simulink model "c28069pmsmfoc_cla"  (R2021b)
settings: Solver=FixedStepDiscrete  StartTime=0.0  StopTime=inf  RelTol=1e-3  EnableMultiTasking=on
PreLoadFcn:
  | c28069pmsmfoc_data;
model workspace (MAT data in the model file):
  encoderResolution = 2000
  hallOffset = '0.5'
  indexOffset = 850
  polePairs = '4'
values from neighbouring files (symbols this model uses):
  Hall_position_offset = 0.57    [c28027pmsmfoc_data.m]    (also in c28035pmsmfoc_data.m; c28035pmsmfoc_data_cla.m; c28069pmsmfoc_data.m)
  PWM_Counter_Period = CPU_frequency/PWM_frequency/2    (= 1500)    [c28027pmsmfoc_data.m]    (also in c28035pmsmfoc_data.m; c28035pmsmfoc_data_cla.m = 2500; c28069pmsmfoc_data.m = 2250)
  Speed_per_unit_scaler = 1200    [c28027pmsmfoc_data.m]    (also in c28035pmsmfoc_data.m; c28035pmsmfoc_data_cla.m = 600; c28069pmsmfoc_data.m)
  Speed_rpm_scaler = 60*CPU_frequency/Pole_pairs/2    (= 450000000)    [c28027pmsmfoc_data.m]    (also in c28035pmsmfoc_data.m; c28035pmsmfoc_data_cla.m; c28069pmsmfoc_data.m = 675000000)
undefined symbols (not defined in the file or in its folder): codertarget, Down, GPTRIP1SEL, GPTRIP2SEL, TZ1, TZ2, Up
libraries: idelinklib_common x12, c2802xlib x7, tiiqmathlib x7, hall_sensor_lib x7, c280xlib x3, c2803xlib x2, simulink x2, etargetslib x2, demo_controls x1, c2806xlib x1, c2000lib x1
(part 1 of 3)
settings Model: Creator=The MathWorks, Inc.  LastModifiedBy=The MathWorks, Inc.
settings SolverCC: AlgebraicLoopSolver=TrustRegion
settings DataIOCC: LimitDataPoints=on  SaveFormat=Array  SaveOutput=off  SaveTime=off  ReturnWorkspaceOutputs=off
settings OptimizationCC: DefaultParameterBehavior=Inlined  DefaultUnderspecifiedDataType=single  InlineInvariantSignals=on  BufferReuse=off  ExpressionDepthLimit=2147483647  InitFltsAndDblsToZero=on  NoFixptDivByZeroProtection=on  EfficientFloat2IntCast=on  EfficientMapNaN2IntZero=off  LifeSpan=Inf  MaxStackSize=512  EfficientTunableParamExpr=on
settings DebuggingCC: ReadBeforeWriteMsg=DisableAll  WriteAfterWriteMsg=DisableAll  WriteAfterReadMsg=DisableAll  AlgebraicLoopMsg=error  ArtificialAlgebraicLoopMsg=error  CheckSSInitialOutputMsg=off  UnderspecifiedInitializationDetection=Classic  MergeDetectMultiDrivingBlocksExec=none  SignalResolutionControl=TryResolveAllWithWarning  SolverPrmCheckMsg=warning  InheritedTsInSrcMsg=none  MultiTaskDSMMsg=none  MultiTaskCondExecSysMsg=none  TasksWithSamePriorityMsg=none  SigSpecEnsureSampleTimeMsg=none  IntegerOverflowMsg=none  ParameterPrecisionLossMsg=none  FcnCallInpInsideContextMsg=warning  AllowSymbolicDim=off  StateNameClashWarn=warning  SFUnexpectedBacktrackingDiag=warning  SFNoUnconditionalDefaultTransitionDiag=warning  SFExecutionAtInitializationDiag=none  SFMachineParentedDataDiag=warning  IntegerSaturationMsg=none  ArithmeticOperatorsInVariantConditions=warning
settings HardwareCC: ProdBitPerChar=16  ProdBitPerInt=16  ProdBitPerPointer=32  ProdBitPerSizeT=32  ProdBitPerPtrDiffT=32  ProdLargestAtomicInteger=Integer  ProdLargestAtomicFloat=None  ProdWordSize=16  ProdHWDeviceType=Texas Instruments->C2000  TargetBitPerChar=16  TargetBitPerInt=16  TargetBitPerPointer=16  TargetLargestAtomicInteger=Integer  TargetIntDivRoundTo=Zero  TargetEndianess=LittleEndian  TargetWordSize=16  TargetHWDeviceType=TI C2000
settings ModelReferenceCC: PropagateSignalLabelsOutOfModel=off
settings SFSimCC: SimUseLocalCustomCode=off  MATLABDynamicMemAlloc=off  CustomCodeUndefinedFunction=UseInterfaceOnly
settings RTWCC: Description=Embedded Coder  SystemTargetFile=ert.tlc  HardwareBoard=TI Piccolo F2806x  TemplateMakefile=ert_default_tmf  GenerateReport=on  RTWUseLocalCustomCode=off  Toolchain=Texas Instruments Code Composer Studio (C2000)  BuildConfiguration=Debug  IncludeHyperlinkInReport=on  LaunchReport=on  GenerateTraceInfo=on  GenerateTraceReport=on  GenerateTraceReportSl=on  GenerateTraceReportSf=on  GenerateTraceReportEml=on
settings CodeAppCC: IgnoreCustomStorageClasses=off  CustomSymbolStrType=$N$R$M  StateflowObjectComments=on  InternalIdentifier=Classic
settings ERTTargetCC: CodeReplacementLibrary=TI C28x  MultiwordLength=2048  ExtModeStaticAllocSize=2048  ConvertIfToSwitch=off  SuppressUnreachableDefaultCases=off
settings ConfigComp: CovMetricSettings=dw  CovSaveCumulativeToWorkspaceVar=on  CovSaveSingleToWorkspaceVar=on  CovExternalEMLEnable=off  CovSFcnEnable=off

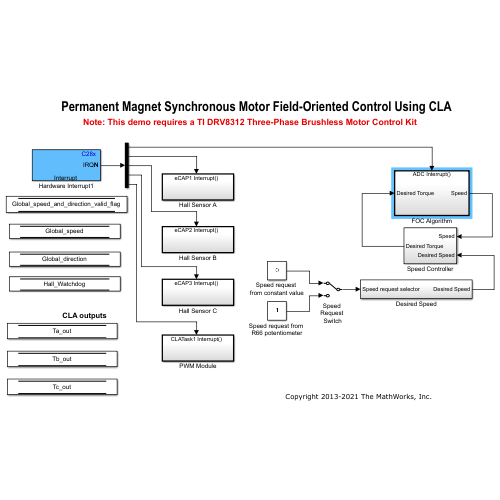
[thumbnail: Simulink's stored preview of the top-level diagram]
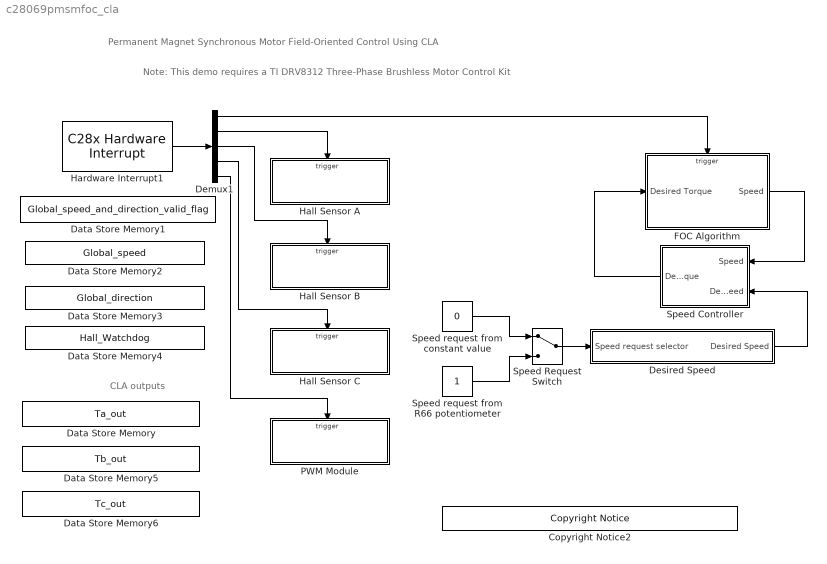
== system c28069pmsmfoc_cla ==
  note: CLA outputs
  note: Note: This demo requires a TI DRV8312 Three-Phase Brushless Motor Control Kit
  note: Permanent Magnet Synchronous Motor Field-Oriented Control Using CLA
  Copyright Notice2 : demo_controls/Copyright Notice  year=2013  prod=tic2000
      settings: SourceProductBaseCode=ME
  Data Store Memory : DataStoreMemory  DataStoreName=Ta_out  ReadBeforeWriteMsg=warning  WriteAfterWriteMsg=warning  WriteAfterReadMsg=warning  EmbeddedSignalClassName=tic2000demospkg.Signal  ShowAdditionalParam=off  OutDataTypeStr=single
  Data Store Memory1 : DataStoreMemory  DataStoreName=Global_speed_and_direction_valid_flag  ReadBeforeWriteMsg=warning  WriteAfterWriteMsg=warning  WriteAfterReadMsg=warning  ShowAdditionalParam=off  OutDataTypeStr=uint16
  Data Store Memory2 : DataStoreMemory  DataStoreName=Global_speed  ReadBeforeWriteMsg=warning  WriteAfterWriteMsg=warning  WriteAfterReadMsg=warning  ShowAdditionalParam=off  OutDataTypeStr=uint32
  Data Store Memory3 : DataStoreMemory  DataStoreName=Global_direction  ReadBeforeWriteMsg=warning  WriteAfterWriteMsg=warning  WriteAfterReadMsg=warning  ShowAdditionalParam=off  OutDataTypeStr=uint16
  Data Store Memory4 : DataStoreMemory  DataStoreName=Hall_Watchdog  ReadBeforeWriteMsg=warning  WriteAfterWriteMsg=warning  WriteAfterReadMsg=warning  InitialValue=65535  ShowAdditionalParam=off  OutDataTypeStr=uint16
  Data Store Memory5 : DataStoreMemory  DataStoreName=Tb_out  ReadBeforeWriteMsg=warning  WriteAfterWriteMsg=warning  WriteAfterReadMsg=warning  EmbeddedSignalClassName=tic2000demospkg.Signal  ShowAdditionalParam=off  OutDataTypeStr=single
  Data Store Memory6 : DataStoreMemory  DataStoreName=Tc_out  ReadBeforeWriteMsg=warning  WriteAfterWriteMsg=warning  WriteAfterReadMsg=warning  EmbeddedSignalClassName=tic2000demospkg.Signal  ShowAdditionalParam=off  OutDataTypeStr=single
  Demux1 : Demux  Outputs=5
  Desired Speed : Subsystem
  FOC Algorithm : Subsystem
  Hall Sensor A : Subsystem  TreatAsAtomicUnit=on
  Hall Sensor B : Subsystem  TreatAsAtomicUnit=on
  Hall Sensor C : Subsystem  TreatAsAtomicUnit=on
  Hardware Interrupt1 : c2000lib/Scheduling/C28x Hardware Interrupt  irqnumbers=[1 4 4 4 11]  pienumbers=[1 1 2 3 1]  irqpriorities=[30 25 25 25 27]  irqpreempts=[1 0 0 0 1]  showinput=off  dspchiptype=C280X
      settings: SourceProductBaseCode=TIC2000
  PWM Module : Subsystem  TreatAsAtomicUnit=on
  Speed Request Switch : ManualSwitch
  Speed Controller : Subsystem
  Speed request from constant value : Constant  Value=0  OutDataTypeStr=uint16
  Speed request from R66 potentiometer : Constant  OutDataTypeStr=uint16
  wires:
  Hardware Interrupt1/1 -> Demux1/1
  Demux1/1 -> FOC Algorithm/Trigger
  Demux1/2 -> Hall Sensor A/Trigger
  Demux1/3 -> Hall Sensor B/Trigger
  Demux1/4 -> Hall Sensor C/Trigger
  FOC Algorithm/1(Speed) -> Speed Controller/1(Speed)
  Speed Controller/1(Desired Torque) -> FOC Algorithm/1(Desired Torque)
  Desired Speed/1(Desired Speed) -> Speed Controller/2(Desired Speed)
  Speed Request Switch/1 -> Desired Speed/1(Speed request selector)
  Speed request from constant value/1 -> Speed Request Switch/1
  Speed request from R66 potentiometer/1 -> Speed Request Switch/2
  Demux1/5 -> PWM Module/Trigger

== system c28069pmsmfoc_cla/Desired Speed ==
  Speed request selector : Inport
  Get_speed_from_R66_potentiometer : Subsystem
  IIR filter : Subsystem
  Per_unit_speed_demand : Constant  Value=+0.5  OutDataTypeStr=fixdt(1,32,17)
      settings: AttributesFormatString=RPM = %<Value> * Speed_per_unit_scaler
  Switch : Switch  Criteria=u2 ~= 0
  Desired Speed : Outport
  wires:
  IIR filter/1(Out1) -> Desired Speed/1
  Switch/1 -> IIR filter/1(In1)
  Get_speed_from_R66_potentiometer/1(Out1) -> Switch/1
  Speed request selector/1 -> Switch/2
  Per_unit_speed_demand/1 -> Switch/3

== system c28069pmsmfoc_cla/FOC Algorithm ==
  Desired Torque : Inport
  ADC Interrupt : TriggerPort  TriggerType=function-call  VariantControl=Variant
  DRV8312 Reset : Constant  Value=ones(1,3)  OutDataTypeStr=uint16  SampleTime=-1
  Digital Output1 : c2803xlib/Digital Output  GPIO_Number=GPIO0~GPIO7  GPIO_Bit0=off  GPIO_BIT0_Toggle=off  GPIO_Bit1=on  GPIO_BIT1_Toggle=off  GPIO_Bit2=off  GPIO_BIT2_Toggle=off  GPIO_Bit3=on  GPIO_BIT3_Toggle=off  GPIO_Bit4=off  GPIO_BIT4_Toggle=off  GPIO_Bit5=on  GPIO_BIT5_Toggle=off  GPIO_Bit6=off  GPIO_BIT6_Toggle=off  GPIO_Bit7=off  GPIO_BIT7_Toggle=off
      settings: SourceProductBaseCode=TIC2000
  IA/IB Measurement : c2802xlib/ADC  blkParamProc=C2000  ADCModule=1  samplingMode=Simultaneous sample mode  ADCResolution=12-bit (Single-ended input)  useSOC1=SOC0  useSOC2=SOC0_SOC1  SOCAcquisitionWindow=7  SOCTriggerSource=ePWM1_ADCSOCA  SOCInterruptTrigger=No ADCINT  Ts=-1  dType=uint16  postInterrupt=on  interruptSel=ADCINT1  ADCINTContinuous=on  endma=off  chdma=1  conv1=ADCINA0  conv2=ADCINA1 and ADCINB1  conv1_Type4=ADCIN0  conv2_Type4=ADCIN0 and ADCIN1
  Torque Control Algorithm : Subsystem
  Speed : Outport  InitialOutput=0
  wires:
  IA/IB Measurement/1 -> Torque Control Algorithm/1(IA/IB)
  DRV8312 Reset/1 -> Digital Output1/1
  Desired Torque/1 -> Torque Control Algorithm/2(Iq_desired)
  Torque Control Algorithm/1(Speed) -> Speed/1

== system c28069pmsmfoc_cla/Hall Sensor A ==
  eCAP1 Interrupt : TriggerPort  TriggerType=function-call  VariantControl=Variant
  Constant2 : Constant  Value=0  OutDataTypeStr=uint16  SampleTime=-1
  Data Store Write2 : DataStoreWrite  DataStoreName=Hall_Watchdog  IndexOptions=Index vector (dialog)  Indices=1  OutputSizes=1
  Demux : Demux  Outputs=2
  Glitch protection : If  IfExpression=u1 > 10000  ShowElse=off
  MinMax : MinMax  Function=max  Inputs=2
  Overflow Detection : Subsystem
  Update Speed and Direction : Subsystem  TreatAsAtomicUnit=on
  eCAP : c280xlib/eCAP  operatingMode=eCAP  selectCAPx=eCAP1  offsetValue=0  counterSynIn=off  enableCounter=off  syncOutput=Disabled  sampleTime=-1  eventPrescaler=0  selectMode=Continuous  enableOneShot=off  stopValue=Capture Event 2  resetEv1Ts=on  ev1Polarity=Rising Edge  resetEv2Ts=on  ev2Polarity=Falling Edge  resetEv3Ts=off  ev3Polarity=Rising Edge  resetEv4Ts=off  ev4Polarity=Rising Edge  tSCntrDataType=uint32  capEvFlag=off  capFlagDataType=uint16  overFlowFlag=on  overFlowFlagDataType=uint16  periodUnit=Seconds  periodSource=Specify via dialog  waveformPeriod=0.001  dutyUnit=Percentages  dutySource=Specify via dialog  dutyCycle=50  outputPolarity=Active High  enableCEVT1Int=on  enableCEVT2Int=on  enableCEVT3Int=off  enableCEVT4Int=off  enableCTROVFInt=on  enablePRDInt=off  enableCMPInt=off
      settings: SourceProductBaseCode=TIC2000
  wires:
  eCAP/1 -> Demux/1, Update Speed and Direction/1(Timers)
  eCAP/2 -> Overflow Detection/1(Overflow_flag)
  Overflow Detection/1(New_local_valid_flag) -> Update Speed and Direction/2(Local_valid_flag)
  Demux/1 -> MinMax/1
  Demux/2 -> MinMax/2
  MinMax/1 -> Glitch protection/1
  Glitch protection/1 -> Update Speed and Direction/Action
  Constant2/1 -> Data Store Write2/1
  Update Speed and Direction/1(New_local_valid_flag) -> Overflow Detection/2(Current_local_valid_flag)

== system c28069pmsmfoc_cla/Hall Sensor B ==
  eCAP2 Interrupt : TriggerPort  TriggerType=function-call  VariantControl=Variant
  Constant2 : Constant  Value=0  OutDataTypeStr=uint16  SampleTime=-1
  Data Store Write2 : DataStoreWrite  DataStoreName=Hall_Watchdog  IndexOptions=Index vector (dialog)  Indices=1  OutputSizes=1
  Demux : Demux  Outputs=2
  Glitch protection : If  IfExpression=u1 > 10000  ShowElse=off
  MinMax : MinMax  Function=max  Inputs=2
  Overflow Detection : Subsystem
  Update Speed and Direction : Subsystem  TreatAsAtomicUnit=on
  eCAP : c280xlib/eCAP  operatingMode=eCAP  selectCAPx=eCAP2  offsetValue=0  counterSynIn=off  enableCounter=off  syncOutput=Disabled  sampleTime=-1  eventPrescaler=0  selectMode=Continuous  enableOneShot=off  stopValue=Capture Event 2  resetEv1Ts=on  ev1Polarity=Rising Edge  resetEv2Ts=on  ev2Polarity=Falling Edge  resetEv3Ts=off  ev3Polarity=Rising Edge  resetEv4Ts=off  ev4Polarity=Rising Edge  tSCntrDataType=uint32  capEvFlag=off  capFlagDataType=uint16  overFlowFlag=on  overFlowFlagDataType=uint16  periodUnit=Seconds  periodSource=Specify via dialog  waveformPeriod=0.001  dutyUnit=Percentages  dutySource=Specify via dialog  dutyCycle=50  outputPolarity=Active High  enableCEVT1Int=on  enableCEVT2Int=on  enableCEVT3Int=off  enableCEVT4Int=off  enableCTROVFInt=on  enablePRDInt=off  enableCMPInt=off
      settings: SourceProductBaseCode=TIC2000
  wires:
  Update Speed and Direction/1(New_local_valid_flag) -> Overflow Detection/2(Current_local_valid_flag)
  Constant2/1 -> Data Store Write2/1
  Glitch protection/1 -> Update Speed and Direction/Action
  MinMax/1 -> Glitch protection/1
  Demux/2 -> MinMax/2
  Demux/1 -> MinMax/1
  Overflow Detection/1(New_local_valid_flag) -> Update Speed and Direction/2(Local_valid_flag)
  eCAP/2 -> Overflow Detection/1(Overflow_flag)
  eCAP/1 -> Update Speed and Direction/1(Timers), Demux/1

== system c28069pmsmfoc_cla/Hall Sensor C ==
  eCAP3 Interrupt : TriggerPort  TriggerType=function-call  VariantControl=Variant
  Constant2 : Constant  Value=0  OutDataTypeStr=uint16  SampleTime=-1
  Data Store Write2 : DataStoreWrite  DataStoreName=Hall_Watchdog  IndexOptions=Index vector (dialog)  Indices=1  OutputSizes=1
  Demux : Demux  Outputs=2
  Glitch protection : If  IfExpression=u1 > 10000  ShowElse=off
  MinMax : MinMax  Function=max  Inputs=2
  Overflow Detection : Subsystem
  Update Speed and Direction : Subsystem  TreatAsAtomicUnit=on
  eCAP : c280xlib/eCAP  operatingMode=eCAP  selectCAPx=eCAP3  offsetValue=0  counterSynIn=off  enableCounter=off  syncOutput=Disabled  sampleTime=-1  eventPrescaler=0  selectMode=Continuous  enableOneShot=off  stopValue=Capture Event 2  resetEv1Ts=on  ev1Polarity=Rising Edge  resetEv2Ts=on  ev2Polarity=Falling Edge  resetEv3Ts=off  ev3Polarity=Rising Edge  resetEv4Ts=off  ev4Polarity=Rising Edge  tSCntrDataType=uint32  capEvFlag=off  capFlagDataType=uint16  overFlowFlag=on  overFlowFlagDataType=uint16  periodUnit=Seconds  periodSource=Specify via dialog  waveformPeriod=0.001  dutyUnit=Percentages  dutySource=Specify via dialog  dutyCycle=50  outputPolarity=Active High  enableCEVT1Int=on  enableCEVT2Int=on  enableCEVT3Int=off  enableCEVT4Int=off  enableCTROVFInt=on  enablePRDInt=off  enableCMPInt=off
      settings: SourceProductBaseCode=TIC2000
  wires:
  eCAP/1 -> Demux/1, Update Speed and Direction/1(Timers)
  eCAP/2 -> Overflow Detection/1(Overflow_flag)
  Overflow Detection/1(New_local_valid_flag) -> Update Speed and Direction/2(Local_valid_flag)
  Demux/1 -> MinMax/1
  Demux/2 -> MinMax/2
  MinMax/1 -> Glitch protection/1
  Glitch protection/1 -> Update Speed and Direction/Action
  Constant2/1 -> Data Store Write2/1
  Update Speed and Direction/1(New_local_valid_flag) -> Overflow Detection/2(Current_local_valid_flag)

== system c28069pmsmfoc_cla/PWM Module ==
  CLATask1 Interrupt : TriggerPort  TriggerType=function-call  VariantControl=Variant
  Data Store Read : DataStoreRead  DataStoreName=Ta_out  IndexOptions=Index vector (dialog)  Indices=1  OutputSizes=1
  Data Store Read1 : DataStoreRead  DataStoreName=Tb_out  IndexOptions=Index vector (dialog)  Indices=1  OutputSizes=1
  Data Store Read2 : DataStoreRead  DataStoreName=Tc_out  IndexOptions=Index vector (dialog)  Indices=1  OutputSizes=1
  Data Type Conversion4 : DataTypeConversion  OutDataTypeStr=fixdt(1,32,17)
  Data Type Conversion5 : DataTypeConversion  OutDataTypeStr=fixdt(1,32,17)
  Data Type Conversion6 : DataTypeConversion  OutDataTypeStr=fixdt(1,32,17)
  Demux : Demux  Outputs=3
  Mux : Mux  Inputs=3
  PWM scaling : Subsystem
  ePWM1 : c2802xlib/ePWM  PwmType=C2000  useModule=ePWM1  ePWMxLINKTBPRD=Not Linked  periodUnits=Clock cycles  timerSource=Specify via dialog  timerPeriod_clk=PWM_Counter_Period+1  timerPeriod_sec=64000  tbshadow=Counter equals to zero  countingMode=Up-Down  phaseActiveEnable=Disable  phaseDirection=Count down after sync  phaseActive=0  synchronizationEnable=off  dcaevt1Sync=off  dcbevt1Sync=off  synchronizationOption=Counter equals to zero (CTR=Zero)  perSynchronizationOption=Counter equals to period (CTR=PRD)  clockPrescale=1  HSclockPrescale=1  enswap=off  ePWMxAStatus=on  ePWMxAactionLogic1=Do nothing  ePWMxAactionLogic2=Do nothing  ePWMxAactionLogic3=Clear  ePWMxAactionLogic4=Set  ePWMxAactionLogic5=Do nothing  ePWMxAactionLogic6=Do nothing  ePWMxACSFenable=off  ePWMxACSFvalue=Forcing disable  ePWMxASFreload=Zero  ePWMxBStatus=off  ePWMxBactionLogic1=Do nothing  ePWMxBactionLogic2=Set  ePWMxBactionLogic3=Do nothing  ePWMxBactionLogic4=Do nothing  ePWMxBactionLogic5=Clear  ePWMxBactionLogic6=Do nothing  ePWMxBCSFenable=off  ePWMxBCSFvalue=Forcing disable  ePWMxBSFreload=Zero  ePWNxBOutWay=off  ePWMxLINKCMPA=Not Linked  CMPAUnits=Clock cycles  CMPASource=Input port  CMPAValue_per=32000  CMPAValue_clk=PWM_Counter_Period/2+1  enCMPAshadow=Counter equals to zero (CTR=Zero)  ePWMxLINKCMPB=Not Linked  CMPBUnits=Clock cycles  CMPBSource=Specify via dialog  CMPBValue_per=50  CMPBValue_clk=PWM_Counter_Period/2+1  enCMPBshadow=Counter equals to zero (CTR=Zero)  ePWMxLINKCMPC=Not Linked  CMPCUnits=Clock cycles  CMPCSource=Specify via dialog  CMPCValue_per=50  CMPCValue_clk=32000  enCMPCshadow=Counter equals to zero (CTR=Zero)  ePWMxLINKCMPD=Not Linked  CMPDUnits=Clock cycles  CMPDSource=Specify via dialog  CMPDValue_per=50  CMPDValue_clk=32000  enCMPDshadow=Counter equals to zero (CTR=Zero)  enableDBePWMxA=off  enableDBePWMxB=off  enhalfcycle=off  DBpolarity=Active high (AH)  DBedgeDelay=Positive  DBSource_ePWMxA=ePWMxA  DBSource_ePWMxB=ePWMxA  DBPeriodUnits=Clock cycles  DBperiodSource=Specify via dialog  REDperiod=0  FEDperiod=0  REDperiod_sec=0  FEDperiod_sec=0  LoadModeDBRED=Immediate without using shadow  LoadModeDBFED=Immediate without using shadow  adcstartModuleA=on  adcrequestEventA=First event  adcstartEventA=Counter equals to period (CTR=PRD)  adcstartEventA_type2=Digital Compare Module A Event 1 start of conversion (DCAEVT1.soc)  adcstartModuleB=off  adcrequestEventB=First event  adcstartEventB=Counter equals to zero (CTR=Zero)  adcstartEventB_type2=Counter equals to zero (CTR=Zero)  intEn=off  intPrd=First event  intSel=Counter equals to zero (CTR=Zero)  intSel_type2=Counter equals to zero (CTR=Zero)  hrpe=off  enHRPWM=off  HRPWM_LoadMode=Counter equals to period (CTR=PRD)  HRPWM_CTLMode=Duty or Period control mode  HRPWM_EDGMode=Both edge  hrpeb=off  enHRPWMB=off  HRPWM_LoadModeB=Counter equals to zero (CTR=ZERO)  HRPWM_CTLModeB=Duty or Period control mode  HRPWM_EDGModeB=Both edge  enHRDBRED=off  enHRDBFED=off  enSFO=on  enautoconv=on  chopperEnable=off  chopperFrequency=1  chopperFirstwidth=1  chopperDuty=12.5%  tripZonesource=Specify via dialog  tzselOSHT1=off  tzselOSHT2=off  tzselOSHT3=off  tzselOSHDCAEV1=off  tzselOSHDCBEV1=off  tzselCBC1=off  tzselCBC2=off  tzselCBC3=off  tzselCBCDCAEV2=off  tzselCBCDCBEV2=off  tzselOSHT4=off  tzselOSHT5=off  tzselOSHT6=off  tzselCBC4=off  tzselCBC5=off  tzselCBC6=off  enTzOstIntr=off  enTzCbcIntr=off  enTzDCAEVT1Intr=off  enTzDCAEVT2Intr=off  enTzDCBEVT1Intr=off  enTzDCBEVT2Intr=off  ePWMxAforced=No action  ePWMxBforced=No action  DCAEVT1forced=No action  DCBEVT1forced=No action  DCAEVT2forced=No action  DCBEVT2forced=No action  dcah=Trip Zone 1 input (TZ1)  dcal=Trip Zone 2 input (TZ2)  dcbh=Trip Zone 1 input (TZ1)  dcbl=Trip Zone 2 input (TZ2)  dcah_type2=GPTRIP1SEL/(TZ1)  dcal_type2=GPTRIP2SEL/(TZ2)  dcbh_type2=GPTRIP1SEL/(TZ1)  dcbl_type2=GPTRIP2SEL/(TZ2)  gendcaevt1=Event disabled  gendcaevt2=Event disabled  gendcbevt1=Event disabled  gendcbevt2=Event disabled  dcaevt1src=DCAEVT1 with sync  dcaevt2src=DCAEVT2 with sync  dcbevt1src=DCBEVT1 with sync  dcbevt2src=DCBEVT2 with sync  pulsesel=Counter equals to zero (CTR=Zero)  blankinv=off  blankoffset=0  blankwidth=0  evsrcsel=Filtered version of DCAEVT1 (DCAEVT1FILT)  encape=off
  ePWM2 : c2802xlib/ePWM  PwmType=C2000  useModule=ePWM2  ePWMxLINKTBPRD=Not Linked  periodUnits=Clock cycles  timerSource=Specify via dialog  timerPeriod_clk=PWM_Counter_Period+1  timerPeriod_sec=64000  tbshadow=Counter equals to zero  countingMode=Up-Down  phaseActiveEnable=Set counter to phase value specified via dialog  phaseDirection=Count up after sync  phaseActive=0  synchronizationEnable=off  dcaevt1Sync=off  dcbevt1Sync=off  synchronizationOption=Pass through (EPWMxSYNCI or SWFSYNC)  perSynchronizationOption=Counter equals to period (CTR=PRD)  clockPrescale=1  HSclockPrescale=1  enswap=off  ePWMxAStatus=on  ePWMxAactionLogic1=Do nothing  ePWMxAactionLogic2=Do nothing  ePWMxAactionLogic3=Clear  ePWMxAactionLogic4=Set  ePWMxAactionLogic5=Do nothing  ePWMxAactionLogic6=Do nothing  ePWMxACSFenable=off  ePWMxACSFvalue=Forcing disable  ePWMxASFreload=Zero  ePWMxBStatus=off  ePWMxBactionLogic1=Do nothing  ePWMxBactionLogic2=Set  ePWMxBactionLogic3=Do nothing  ePWMxBactionLogic4=Do nothing  ePWMxBactionLogic5=Clear  ePWMxBactionLogic6=Do nothing  ePWMxBCSFenable=off  ePWMxBCSFvalue=Forcing disable  ePWMxBSFreload=Zero  ePWNxBOutWay=off  ePWMxLINKCMPA=Not Linked  CMPAUnits=Clock cycles  CMPASource=Input port  CMPAValue_per=32000  CMPAValue_clk=PWM_Counter_Period/2+1  enCMPAshadow=Counter equals to zero (CTR=Zero)  ePWMxLINKCMPB=Not Linked  CMPBUnits=Clock cycles  CMPBSource=Specify via dialog  CMPBValue_per=50  CMPBValue_clk=PWM_Counter_Period/2+1  enCMPBshadow=Counter equals to zero (CTR=Zero)  ePWMxLINKCMPC=Not Linked  CMPCUnits=Clock cycles  CMPCSource=Specify via dialog  CMPCValue_per=50  CMPCValue_clk=32000  enCMPCshadow=Counter equals to zero (CTR=Zero)  ePWMxLINKCMPD=Not Linked  CMPDUnits=Clock cycles  CMPDSource=Specify via dialog  CMPDValue_per=50  CMPDValue_clk=32000  enCMPDshadow=Counter equals to zero (CTR=Zero)  enableDBePWMxA=off  enableDBePWMxB=off  enhalfcycle=off  DBpolarity=Active high (AH)  DBedgeDelay=Positive  DBSource_ePWMxA=ePWMxA  DBSource_ePWMxB=ePWMxA  DBPeriodUnits=Clock cycles  DBperiodSource=Specify via dialog  REDperiod=0  FEDperiod=0  REDperiod_sec=0  FEDperiod_sec=0  LoadModeDBRED=Immediate without using shadow  LoadModeDBFED=Immediate without using shadow  adcstartModuleA=off  adcrequestEventA=First event  adcstartEventA=Digital Compare Module A Event 1 start of conversion (DCAEVT1.soc)  adcstartEventA_type2=Digital Compare Module A Event 1 start of conversion (DCAEVT1.soc)  adcstartModuleB=off  adcrequestEventB=First event  adcstartEventB=Counter equals to zero (CTR=Zero)  adcstartEventB_type2=Counter equals to zero (CTR=Zero)  intEn=off  intPrd=First event  intSel=Counter equals to zero (CTR=Zero)  intSel_type2=Counter equals to zero (CTR=Zero)  hrpe=off  enHRPWM=off  HRPWM_LoadMode=Counter equals to period (CTR=PRD)  HRPWM_CTLMode=Duty or Period control mode  HRPWM_EDGMode=Both edge  hrpeb=off  enHRPWMB=off  HRPWM_LoadModeB=Counter equals to zero (CTR=ZERO)  HRPWM_CTLModeB=Duty or Period control mode  HRPWM_EDGModeB=Both edge  enHRDBRED=off  enHRDBFED=off  enSFO=on  enautoconv=on  chopperEnable=off  chopperFrequency=1  chopperFirstwidth=1  chopperDuty=12.5%  tripZonesource=Specify via dialog  tzselOSHT1=off  tzselOSHT2=off  tzselOSHT3=off  tzselOSHDCAEV1=off  tzselOSHDCBEV1=off  tzselCBC1=off  tzselCBC2=off  tzselCBC3=off  tzselCBCDCAEV2=off  tzselCBCDCBEV2=off  tzselOSHT4=off  tzselOSHT5=off  tzselOSHT6=off  tzselCBC4=off  tzselCBC5=off  tzselCBC6=off  enTzOstIntr=off  enTzCbcIntr=off  enTzDCAEVT1Intr=off  enTzDCAEVT2Intr=off  enTzDCBEVT1Intr=off  enTzDCBEVT2Intr=off  ePWMxAforced=No action  ePWMxBforced=No action  DCAEVT1forced=No action  DCBEVT1forced=No action  DCAEVT2forced=No action  DCBEVT2forced=No action  dcah=Trip Zone 1 input (TZ1)  dcal=Trip Zone 2 input (TZ2)  dcbh=Trip Zone 1 input (TZ1)  dcbl=Trip Zone 2 input (TZ2)  dcah_type2=GPTRIP1SEL/(TZ1)  dcal_type2=GPTRIP2SEL/(TZ2)  dcbh_type2=GPTRIP1SEL/(TZ1)  dcbl_type2=GPTRIP2SEL/(TZ2)  gendcaevt1=Event disabled  gendcaevt2=Event disabled  gendcbevt1=Event disabled  gendcbevt2=Event disabled  dcaevt1src=DCAEVT1 with sync  dcaevt2src=DCAEVT2 with sync  dcbevt1src=DCBEVT1 with sync  dcbevt2src=DCBEVT2 with sync  pulsesel=Counter equals to zero (CTR=Zero)  blankinv=off  blankoffset=0  blankwidth=0  evsrcsel=Filtered version of DCAEVT1 (DCAEVT1FILT)  encape=off
  ePWM3 : c2802xlib/ePWM  PwmType=C2000  useModule=ePWM3  ePWMxLINKTBPRD=Not Linked  periodUnits=Clock cycles  timerSource=Specify via dialog  timerPeriod_clk=PWM_Counter_Period+1  timerPeriod_sec=64000  tbshadow=Counter equals to zero  countingMode=Up-Down  phaseActiveEnable=Set counter to phase value specified via dialog  phaseDirection=Count up after sync  phaseActive=0  synchronizationEnable=off  dcaevt1Sync=off  dcbevt1Sync=off  synchronizationOption=Disable  perSynchronizationOption=Counter equals to period (CTR=PRD)  clockPrescale=1  HSclockPrescale=1  enswap=off  ePWMxAStatus=on  ePWMxAactionLogic1=Do nothing  ePWMxAactionLogic2=Do nothing  ePWMxAactionLogic3=Clear  ePWMxAactionLogic4=Set  ePWMxAactionLogic5=Do nothing  ePWMxAactionLogic6=Do nothing  ePWMxACSFenable=off  ePWMxACSFvalue=Forcing disable  ePWMxASFreload=Zero  ePWMxBStatus=off  ePWMxBactionLogic1=Do nothing  ePWMxBactionLogic2=Set  ePWMxBactionLogic3=Do nothing  ePWMxBactionLogic4=Do nothing  ePWMxBactionLogic5=Clear  ePWMxBactionLogic6=Do nothing  ePWMxBCSFenable=off  ePWMxBCSFvalue=Forcing disable  ePWMxBSFreload=Zero  ePWNxBOutWay=off  ePWMxLINKCMPA=Not Linked  CMPAUnits=Clock cycles  CMPASource=Input port  CMPAValue_per=32000  CMPAValue_clk=PWM_Counter_Period/2+1  enCMPAshadow=Counter equals to zero (CTR=Zero)  ePWMxLINKCMPB=Not Linked  CMPBUnits=Clock cycles  CMPBSource=Specify via dialog  CMPBValue_per=50  CMPBValue_clk=PWM_Counter_Period/2+1  enCMPBshadow=Counter equals to zero (CTR=Zero)  ePWMxLINKCMPC=Not Linked  CMPCUnits=Clock cycles  CMPCSource=Specify via dialog  CMPCValue_per=50  CMPCValue_clk=32000  enCMPCshadow=Counter equals to zero (CTR=Zero)  ePWMxLINKCMPD=Not Linked  CMPDUnits=Clock cycles  CMPDSource=Specify via dialog  CMPDValue_per=50  CMPDValue_clk=32000  enCMPDshadow=Counter equals to zero (CTR=Zero)  enableDBePWMxA=off  enableDBePWMxB=off  enhalfcycle=off  DBpolarity=Active high (AH)  DBedgeDelay=Positive  DBSource_ePWMxA=ePWMxA  DBSource_ePWMxB=ePWMxA  DBPeriodUnits=Clock cycles  DBperiodSource=Specify via dialog  REDperiod=0  FEDperiod=0  REDperiod_sec=0  FEDperiod_sec=0  LoadModeDBRED=Immediate without using shadow  LoadModeDBFED=Immediate without using shadow  adcstartModuleA=off  adcrequestEventA=First event  adcstartEventA=Digital Compare Module A Event 1 start of conversion (DCAEVT1.soc)  adcstartEventA_type2=Digital Compare Module A Event 1 start of conversion (DCAEVT1.soc)  adcstartModuleB=off  adcrequestEventB=First event  adcstartEventB=Counter equals to zero (CTR=Zero)  adcstartEventB_type2=Counter equals to zero (CTR=Zero)  intEn=off  intPrd=First event  intSel=Counter equals to zero (CTR=Zero)  intSel_type2=Counter equals to zero (CTR=Zero)  hrpe=off  enHRPWM=off  HRPWM_LoadMode=Counter equals to period (CTR=PRD)  HRPWM_CTLMode=Duty or Period control mode  HRPWM_EDGMode=Both edge  hrpeb=off  enHRPWMB=off  HRPWM_LoadModeB=Counter equals to zero (CTR=ZERO)  HRPWM_CTLModeB=Duty or Period control mode  HRPWM_EDGModeB=Both edge  enHRDBRED=off  enHRDBFED=off  enSFO=on  enautoconv=on  chopperEnable=off  chopperFrequency=1  chopperFirstwidth=1  chopperDuty=12.5%  tripZonesource=Specify via dialog  tzselOSHT1=off  tzselOSHT2=off  tzselOSHT3=off  tzselOSHDCAEV1=off  tzselOSHDCBEV1=off  tzselCBC1=off  tzselCBC2=off  tzselCBC3=off  tzselCBCDCAEV2=off  tzselCBCDCBEV2=off  tzselOSHT4=off  tzselOSHT5=off  tzselOSHT6=off  tzselCBC4=off  tzselCBC5=off  tzselCBC6=off  enTzOstIntr=off  enTzCbcIntr=off  enTzDCAEVT1Intr=off  enTzDCAEVT2Intr=off  enTzDCBEVT1Intr=off  enTzDCBEVT2Intr=off  ePWMxAforced=No action  ePWMxBforced=No action  DCAEVT1forced=No action  DCBEVT1forced=No action  DCAEVT2forced=No action  DCBEVT2forced=No action  dcah=Trip Zone 1 input (TZ1)  dcal=Trip Zone 2 input (TZ2)  dcbh=Trip Zone 1 input (TZ1)  dcbl=Trip Zone 2 input (TZ2)  dcah_type2=GPTRIP1SEL/(TZ1)  dcal_type2=GPTRIP2SEL/(TZ2)  dcbh_type2=GPTRIP1SEL/(TZ1)  dcbl_type2=GPTRIP2SEL/(TZ2)  gendcaevt1=Event disabled  gendcaevt2=Event disabled  gendcbevt1=Event disabled  gendcbevt2=Event disabled  dcaevt1src=DCAEVT1 with sync  dcaevt2src=DCAEVT2 with sync  dcbevt1src=DCBEVT1 with sync  dcbevt2src=DCBEVT2 with sync  pulsesel=Counter equals to zero (CTR=Zero)  blankinv=off  blankoffset=0  blankwidth=0  evsrcsel=Filtered version of DCAEVT1 (DCAEVT1FILT)  encape=off
  wires:
  Data Store Read/1 -> Data Type Conversion4/1
  Data Store Read1/1 -> Data Type Conversion5/1
  Data Store Read2/1 -> Data Type Conversion6/1
  PWM scaling/1(PWM A/B/C) -> Demux/1
  Mux/1 -> PWM scaling/1(Ta/Tb/Tc)
  Demux/1 -> ePWM1/1
  Demux/2 -> ePWM2/1
  Demux/3 -> ePWM3/1
  Data Type Conversion4/1 -> Mux/1
  Data Type Conversion5/1 -> Mux/2
  Data Type Conversion6/1 -> Mux/3

== system c28069pmsmfoc_cla/Speed Controller ==
  Speed : Inport
  Desired Speed : Inport  Port=2
  PID Controller : Subsystem  InitFcn=|  mask(PID Controller){proportionalGain=0.04, integralGain=0.1, correctionGain=0.1, derivativeGain=0, minOutput=-1, maxOutput=1}
      | tic2000lib_licenseCheck;
      | codertarget.registry.registerC28xNonPeripheralBlocks(gcb);
      mask prompts: proportionalGain "Proportional gain:"; integralGain "Integral gain:"; correctionGain "Integral correction gain:"; derivativeGain "Derivative gain:"; minOutput "Minimum output:"; maxOutput "Maximum output:"
      mask help: This block implements a digital PID controller with anti-windup correction. Both inputs and the output are signed 32-bit fixed-point numbers with Q value between 1 and 29.
      mask init:
      | c280xDMCPIDControl_callback(proportionalGain,integralGain,correctionGain,derivativeGain,minOutput,maxOutput)
      mask Help: eval('codertarget.internal.helpView(''tic2000'' ,''c28xdmclibpidcontroller'')')
      mask Display:
      | port_label('input',1,'ref');
      | port_label('input',2,'fdb');
      | port_label('Output',1,'out');
      | text(0.5,0.15, 'PID', 'horizontalalignment','center');
  Rate Transition : RateTransition  Integrity=off  OutPortSampleTime=0.01
  Rate Transition1 : RateTransition  Integrity=off
  Send to DAC 1/2 : Subsystem
  Desired Torque : Outport
  wires:
  PID Controller/1(Out1) -> Send to DAC 1/2/2(IQ_desired), Rate Transition1/1
  Desired Speed/1 -> PID Controller/1(In1)
  Rate Transition/1 -> Send to DAC 1/2/1(speed), PID Controller/2(In2)
  Speed/1 -> Rate Transition/1
  Rate Transition1/1 -> Desired Torque/1

== system c28069pmsmfoc_cla/Desired Speed/Get_speed_from_R66_potentiometer ==
  ADC : c2802xlib/ADC  blkParamProc=C2000  ADCModule=1  samplingMode=Single sample mode  ADCResolution=12-bit (Single-ended input)  useSOC1=SOC2  useSOC2=SOC0_SOC1  SOCAcquisitionWindow=7  SOCTriggerSource=Software  SOCInterruptTrigger=No ADCINT  Ts=-1  dType=uint16  postInterrupt=off  interruptSel=ADCINT1  ADCINTContinuous=off  endma=off  chdma=1  conv1=ADCINB0  conv2=ADCINA0 and ADCINB0  conv1_Type4=ADCIN0  conv2_Type4=ADCIN0 and ADCIN1
  Add2 : Sum  Inputs=+-
  Constant2 : Constant  Value=.1  OutDataTypeStr=fixdt(1,32,17)
  Data Type Conversion1 : DataTypeConversion  OutDataTypeStr=fixdt(1,32,17)  ConvertRealWorld=Stored Integer (SI)
  Saturation1 : Saturate  UpperLimit=1  LowerLimit=0
  Shift Arithmetic1 : ArithShift  BitShiftNumber=-5
  Out1 : Outport
  wires:
  Data Type Conversion1/1 -> Shift Arithmetic1/1
  ADC/1 -> Data Type Conversion1/1
  Add2/1 -> Saturation1/1
  Constant2/1 -> Add2/2
  Shift Arithmetic1/1 -> Add2/1
  Saturation1/1 -> Out1/1

== system c28069pmsmfoc_cla/Desired Speed/IIR filter ==
  In1 : Inport
  Add : Sum  Inputs=+-
  Add1 : Sum
  Constant : Constant  OutDataTypeStr=fixdt(1,32,17)
  Constant1 : Constant  Value=.04  OutDataTypeStr=fixdt(1,32,17)
  IQN x IQN : tiiqmathlib/IQN x IQN  multiplyOption=Multiply
      settings: SourceProductBaseCode=TIC2000
  IQN x IQN1 : tiiqmathlib/IQN x IQN  multiplyOption=Multiply
      settings: SourceProductBaseCode=TIC2000
  Unit Delay : UnitDelay  SampleTime=-1  HasFrameUpgradeWarning=on
  Out1 : Outport
  wires:
  IQN x IQN1/1 -> Add1/2
  Unit Delay/1 -> IQN x IQN1/2
  Add/1 -> IQN x IQN1/1
  IQN x IQN/1 -> Add1/1
  Constant1/1 -> IQN x IQN/2, Add/2
  Constant/1 -> Add/1
  Add1/1 -> Out1/1, Unit Delay/1
  In1/1 -> IQN x IQN/1

== system c28069pmsmfoc_cla/FOC Algorithm/Torque Control Algorithm ==
  IA/IB : Inport
  Iq_desired : Inport  Port=2
  Atomic Hall Reading : Subsystem  TreatAsAtomicUnit=on
      settings: RTWSystemCode=Nonreusable function
  Direction LED GPIO34 : c2803xlib/Digital Output  GPIO_Number=GPIO32~GPIO39  GPIO_Bit0=off  GPIO_BIT0_Toggle=off  GPIO_Bit1=off  GPIO_BIT1_Toggle=off  GPIO_Bit2=on  GPIO_BIT2_Toggle=off  GPIO_Bit3=off  GPIO_BIT3_Toggle=off  GPIO_Bit4=off  GPIO_BIT4_Toggle=off  GPIO_Bit5=off  GPIO_BIT5_Toggle=off  GPIO_Bit6=off  GPIO_BIT6_Toggle=off  GPIO_Bit7=off  GPIO_BIT7_Toggle=off
      settings: SourceProductBaseCode=TIC2000
  Direction Scaling : Subsystem
  Generating Space Vectors : Subsystem
  Input Scaling : Subsystem
  Selector1 : Selector  InputPortWidth=3  IndexOptions=Index vector (dialog)  Indices=[1]  OutputSizes=1
  Selector2 : Selector  InputPortWidth=3  IndexOptions=Index vector (dialog)  Indices=3  OutputSizes=1
  Selector3 : Selector  InputPortWidth=3  IndexOptions=Index vector (dialog)  Indices=2  OutputSizes=1
  Send to DAC 3 : Subsystem
  Speed IIR filter : Subsystem
  Speed : Outport
  wires:
  Atomic Hall Reading/1(Direction) -> Input Scaling/1(Dir)
  Atomic Hall Reading/2(Valid Flag) -> Input Scaling/2(Valid Flag)
  Atomic Hall Reading/3(Speed) -> Input Scaling/3(speed counts)
  Atomic Hall Reading/4(Halls) -> Input Scaling/4(Halls)
  Atomic Hall Reading/5(Hall Watchdog) -> Input Scaling/5(Hall_Watchdog)
  Input Scaling/1(Dir/Pos/Speed) -> Generating Space Vectors/1(Speed/Pos/Dir), Selector2/1, Selector3/1, Selector1/1
  Direction Scaling/1(Binary Direction) -> Direction LED GPIO34/1
  IA/IB/1 -> Input Scaling/6(IA/IB)
  Input Scaling/3(Ib) -> Generating Space Vectors/3(Ib)
  Input Scaling/2(Ia) -> Generating Space Vectors/2(Ia)
  Iq_desired/1 -> Generating Space Vectors/4(Iq Desired)
  Selector1/1 -> Direction Scaling/1(Dir)
  Selector2/1 -> Speed IIR filter/1(Speed)
  Speed IIR filter/1(Filtered speed) -> Speed/1
  Selector3/1 -> Send to DAC 3/1(Position)

== system c28069pmsmfoc_cla/Hall Sensor A/Overflow Detection ==
  note: The overflow detection will reset the global speed and direction valid flag
  Overflow_flag : Inport
  Current_local_valid_flag : Inport  Port=2
  Detects an overflow of the eCAP counter : If  IfExpression=u1 ~= 0
  Merge : Merge
  No overflow detected : Subsystem
  Overflow detected : Subsystem  TreatAsAtomicUnit=on
  New_local_valid_flag : Outport
  wires:
  Detects an overflow of the eCAP counter/2 -> No overflow detected/Action
  Detects an overflow of the eCAP counter/1 -> Overflow detected/Action
  Overflow_flag/1 -> Detects an overflow of the eCAP counter/1
  Current_local_valid_flag/1 -> No overflow detected/1(old_validate)
  Overflow detected/1(New_valid_flag) -> Merge/1
  No overflow detected/1(New_valid_flag) -> Merge/2
  Merge/1 -> New_local_valid_flag/1

== system c28069pmsmfoc_cla/Hall Sensor A/Update Speed and Direction ==
  Timers : Inport
  Local_valid_flag : Inport  Port=2
  Action Port : ActionPort  ActionPortLabel=if(u1 > 10000)
  Hall Step : hall_sensor_lib/Hall step  hallRisingDir0=5  hallRisingDir1=3  hallFallingDir0=2  hallFallingDir1=4
      settings: SourceProductBaseCode=TIC2000
  If : If  IfExpression=u1 ~= 0  ShowElse=off
  Read Global Direction : DataStoreRead  DataStoreName=Global_direction  IndexOptions=Index vector (dialog)  Indices=1  OutputSizes=1
  Read_halls : hall_sensor_lib/Read_halls  sample_time=-1
      settings: SourceProductBaseCode=TIC2000
  Update Global Direction : DataStoreWrite  DataStoreName=Global_direction  IndexOptions=Index vector (dialog)  Indices=1  OutputSizes=1
  Update Global Speed and Direction Valid Flag : DataStoreWrite  DataStoreName=Global_speed_and_direction_valid_flag  IndexOptions=Index vector (dialog)  Indices=1  OutputSizes=1
  update_speed : Subsystem
  New_local_valid_flag : Outport
  wires:
  Hall Step/3 -> Update Global Speed and Direction Valid Flag/1, If/1
  Hall Step/1 -> New_local_valid_flag/1
  If/1 -> update_speed/Action
  Hall Step/2 -> Update Global Direction/1
  Read Global Direction/1 -> Hall Step/2
  Local_valid_flag/1 -> Hall Step/3
  Read_halls/1 -> Hall Step/1
  Timers/1 -> Hall Step/4
  Hall Step/4 -> update_speed/1(In1)

== system c28069pmsmfoc_cla/Hall Sensor B/Overflow Detection ==
  note: The overflow detection will reset the global speed and direction valid flag
  Overflow_flag : Inport
  Current_local_valid_flag : Inport  Port=2
  Detects an overflow of the eCAP counter : If  IfExpression=u1 ~= 0
  Merge : Merge
  No overflow detected : Subsystem
  Overflow detected : Subsystem  TreatAsAtomicUnit=on
  New_local_valid_flag : Outport
  wires:
  Merge/1 -> New_local_valid_flag/1
  No overflow detected/1(New_valid_flag) -> Merge/2
  Overflow detected/1(New_valid_flag) -> Merge/1
  Current_local_valid_flag/1 -> No overflow detected/1(old_validate)
  Overflow_flag/1 -> Detects an overflow of the eCAP counter/1
  Detects an overflow of the eCAP counter/1 -> Overflow detected/Action
  Detects an overflow of the eCAP counter/2 -> No overflow detected/Action

== system c28069pmsmfoc_cla/Hall Sensor B/Update Speed and Direction ==
  Timers : Inport
  Local_valid_flag : Inport  Port=2
  Action Port : ActionPort  ActionPortLabel=if(u1 > 10000)
  Hall Step : hall_sensor_lib/Hall step  hallRisingDir0=3  hallRisingDir1=6  hallFallingDir0=4  hallFallingDir1=1
      settings: SourceProductBaseCode=TIC2000
  If : If  IfExpression=u1 ~= 0  ShowElse=off
  Read Global Direction : DataStoreRead  DataStoreName=Global_direction  IndexOptions=Index vector (dialog)  Indices=1  OutputSizes=1
  Read_halls : hall_sensor_lib/Read_halls  sample_time=-1
      settings: SourceProductBaseCode=TIC2000
  Update Global Direction : DataStoreWrite  DataStoreName=Global_direction  IndexOptions=Index vector (dialog)  Indices=1  OutputSizes=1
  Update Global Speed and Direction Valid Flag : DataStoreWrite  DataStoreName=Global_speed_and_direction_valid_flag  IndexOptions=Index vector (dialog)  Indices=1  OutputSizes=1
  update_speed : Subsystem
  New_local_valid_flag : Outport
  wires:
  Hall Step/4 -> update_speed/1(In1)
  Timers/1 -> Hall Step/4
  Read_halls/1 -> Hall Step/1
  Local_valid_flag/1 -> Hall Step/3
  Read Global Direction/1 -> Hall Step/2
  Hall Step/2 -> Update Global Direction/1
  If/1 -> update_speed/Action
  Hall Step/1 -> New_local_valid_flag/1
  Hall Step/3 -> If/1, Update Global Speed and Direction Valid Flag/1

== system c28069pmsmfoc_cla/Hall Sensor C/Overflow Detection ==
  note: The overflow detection will reset the global speed and direction valid flag
  Overflow_flag : Inport
  Current_local_valid_flag : Inport  Port=2
  Detects an overflow of the eCAP counter : If  IfExpression=u1 ~= 0
  Merge : Merge
  No overflow detected : Subsystem
  Overflow detected : Subsystem  TreatAsAtomicUnit=on
  New_local_valid_flag : Outport
  wires:
  Detects an overflow of the eCAP counter/2 -> No overflow detected/Action
  Detects an overflow of the eCAP counter/1 -> Overflow detected/Action
  Overflow_flag/1 -> Detects an overflow of the eCAP counter/1
  Current_local_valid_flag/1 -> No overflow detected/1(old_validate)
  Overflow detected/1(New_valid_flag) -> Merge/1
  No overflow detected/1(New_valid_flag) -> Merge/2
  Merge/1 -> New_local_valid_flag/1

== system c28069pmsmfoc_cla/Hall Sensor C/Update Speed and Direction ==
  Timers : Inport
  Local_valid_flag : Inport  Port=2
  Action Port : ActionPort  ActionPortLabel=if(u1 > 10000)
  Hall Step1 : hall_sensor_lib/Hall step  hallRisingDir0=6  hallRisingDir1=5  hallFallingDir0=1  hallFallingDir1=2
      settings: SourceProductBaseCode=TIC2000
  If : If  IfExpression=u1 ~= 0  ShowElse=off
  Read Global Direction : DataStoreRead  DataStoreName=Global_direction  IndexOptions=Index vector (dialog)  Indices=1  OutputSizes=1
  Read_halls : hall_sensor_lib/Read_halls  sample_time=-1
      settings: SourceProductBaseCode=TIC2000
  Update Global Direction : DataStoreWrite  DataStoreName=Global_direction  IndexOptions=Index vector (dialog)  Indices=1  OutputSizes=1
  Update Global Speed and Direction Valid Flag : DataStoreWrite  DataStoreName=Global_speed_and_direction_valid_flag  IndexOptions=Index vector (dialog)  Indices=1  OutputSizes=1
  update_speed : Subsystem
  New_local_valid_flag : Outport
  wires:
  Hall Step1/3 -> Update Global Speed and Direction Valid Flag/1, If/1
  Hall Step1/1 -> New_local_valid_flag/1
  If/1 -> update_speed/Action
  Hall Step1/2 -> Update Global Direction/1
  Read Global Direction/1 -> Hall Step1/2
  Local_valid_flag/1 -> Hall Step1/3
  Read_halls/1 -> Hall Step1/1
  Timers/1 -> Hall Step1/4
  Hall Step1/4 -> update_speed/1(In1)

== system c28069pmsmfoc_cla/PWM Module/PWM scaling ==
  Ta/Tb/Tc : Inport
  Add : Sum
  Constant : Constant  OutDataTypeStr=fixdt(1,32,17)
  Data Type Conversion : DataTypeConversion  OutDataTypeStr=uint16
  PWM_Counter_Period : Gain  Gain=PWM_Counter_Period/2  ParamDataTypeStr=fixdt(1,32,2)  OutDataTypeStr=fixdt(1,32,2)
  PWM A/B/C : Outport
  wires:
  Constant/1 -> Add/1
  Add/1 -> PWM_Counter_Period/1
  Ta/Tb/Tc/1 -> Add/2
  PWM_Counter_Period/1 -> Data Type Conversion/1
  Data Type Conversion/1 -> PWM A/B/C/1

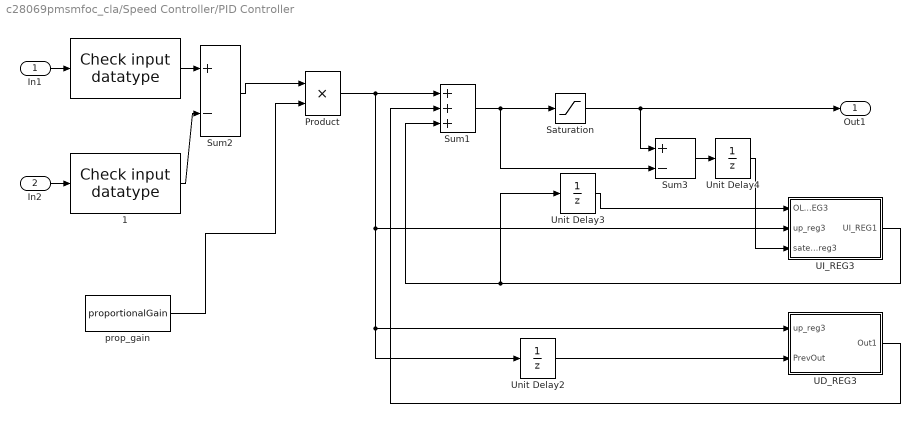
== system c28069pmsmfoc_cla/Speed Controller/PID Controller ==
  In1 : Inport
  In2 : Inport  Port=2
  " " : etargetslib/ 
      settings: SourceProductBaseCode=ME
  " 1" : etargetslib/ 
      settings: SourceProductBaseCode=ME
  Product : Product  OutDataTypeStr=Inherit: Same as first input
  Saturation : Saturate  UpperLimit=maxOutput  LowerLimit=minOutput  LinearizeAsGain=off  ZeroCross=off
  Sum1 : Sum  Inputs=+++
  Sum2 : Sum  Inputs=+-
  Sum3 : Sum  Inputs=+-
  UD_REG3 : Subsystem
  UI_REG3 : Subsystem
  Unit Delay2 : UnitDelay  SampleTime=-1  HasFrameUpgradeWarning=on
  Unit Delay3 : UnitDelay  SampleTime=-1  HasFrameUpgradeWarning=on
  Unit Delay4 : UnitDelay  SampleTime=-1  HasFrameUpgradeWarning=on
  prop_gain : Constant  Value=proportionalGain  OutDataTypeStr=Inherit: Inherit via back propagation
  Out1 : Outport
  wires:
  " 1"/1 -> Sum2/2
  " "/1 -> Sum2/1
  prop_gain/1 -> Product/2
  Unit Delay2/1 -> UD_REG3/2(PrevOut)
  Sum3/1 -> Unit Delay4/1
  Saturation/1 -> Out1/1, Sum3/1
  Sum1/1 -> Sum3/2, Saturation/1
  UI_REG3/1(UI_REG1) -> Sum1/3, Unit Delay3/1
  UD_REG3/1(Out1) -> Sum1/2
  Product/1 -> Unit Delay2/1, UD_REG3/1(up_reg3), UI_REG3/2(up_reg3), Sum1/1
  Sum2/1 -> Product/1
  In2/1 -> " 1"/1
  In1/1 -> " "/1
  Unit Delay3/1 -> UI_REG3/1(OLD_UI_REG3)
  Unit Delay4/1 -> UI_REG3/3(saterr_reg3)

== system c28069pmsmfoc_cla/Speed Controller/Send to DAC 1//2 ==
  speed : Inport
  IQ_desired : Inport  Port=2
  Bias1 : Bias  Bias=1
  Bias2 : Bias  Bias=1
  Bitwise Operator : simulink/Logic and Bit Operations/Bitwise Operator  logicop=AND  UseBitMask=on  BitMask=hex2dec('0FFF')  BitMaskRealWorld=Stored Integer
  Data Type Conversion : DataTypeConversion  OutDataTypeStr=uint16  ConvertRealWorld=Stored Integer (SI)
  Demux : Demux  Outputs=2
  Mux : Mux  Inputs=2
  Shift Arithmetic : ArithShift  BitShiftNumber=6  BitShiftDirection=Right
  Shift Arithmetic1 : ArithShift  BitShiftNumber=6  BitShiftDirection=Right
  ePWM2 : c2802xlib/ePWM  PwmType=C2000  useModule=ePWM6  ePWMxLINKTBPRD=Not Linked  periodUnits=Clock cycles  timerSource=Specify via dialog  timerPeriod_clk=4097  timerPeriod_sec=64000  tbshadow=Counter equals to zero  countingMode=Up  phaseActiveEnable=Disable  phaseDirection=Count down after sync  phaseActive=0  synchronizationEnable=off  dcaevt1Sync=off  dcbevt1Sync=off  synchronizationOption=Disable  perSynchronizationOption=Counter equals to period (CTR=PRD)  clockPrescale=1  HSclockPrescale=1  enswap=off  ePWMxAStatus=on  ePWMxAactionLogic1=Do nothing  ePWMxAactionLogic2=Set  ePWMxAactionLogic3=Clear  ePWMxAactionLogic4=Do nothing  ePWMxAactionLogic5=Do nothing  ePWMxAactionLogic6=Do nothing  ePWMxACSFenable=off  ePWMxACSFvalue=Forcing disable  ePWMxASFreload=Zero  ePWMxBStatus=on  ePWMxBactionLogic1=Do nothing  ePWMxBactionLogic2=Set  ePWMxBactionLogic3=Do nothing  ePWMxBactionLogic4=Do nothing  ePWMxBactionLogic5=Clear  ePWMxBactionLogic6=Do nothing  ePWMxBCSFenable=off  ePWMxBCSFvalue=Forcing disable  ePWMxBSFreload=Zero  ePWNxBOutWay=off  ePWMxLINKCMPA=Not Linked  CMPAUnits=Clock cycles  CMPASource=Input port  CMPAValue_per=32000  CMPAValue_clk=0  enCMPAshadow=Counter equals to zero (CTR=Zero)  ePWMxLINKCMPB=Not Linked  CMPBUnits=Clock cycles  CMPBSource=Input port  CMPBValue_per=50  CMPBValue_clk=0  enCMPBshadow=Counter equals to zero (CTR=Zero)  ePWMxLINKCMPC=Not Linked  CMPCUnits=Clock cycles  CMPCSource=Specify via dialog  CMPCValue_per=50  CMPCValue_clk=32000  enCMPCshadow=Counter equals to zero (CTR=Zero)  ePWMxLINKCMPD=Not Linked  CMPDUnits=Clock cycles  CMPDSource=Specify via dialog  CMPDValue_per=50  CMPDValue_clk=32000  enCMPDshadow=Counter equals to zero (CTR=Zero)  enableDBePWMxA=off  enableDBePWMxB=off  enhalfcycle=off  DBpolarity=Active high (AH)  DBedgeDelay=Positive  DBSource_ePWMxA=ePWMxA  DBSource_ePWMxB=ePWMxA  DBPeriodUnits=Clock cycles  DBperiodSource=Specify via dialog  REDperiod=0  FEDperiod=0  REDperiod_sec=0  FEDperiod_sec=0  LoadModeDBRED=Immediate without using shadow  LoadModeDBFED=Immediate without using shadow  adcstartModuleA=off  adcrequestEventA=First event  adcstartEventA=Digital Compare Module A Event 1 start of conversion (DCAEVT1.soc)  adcstartEventA_type2=Digital Compare Module A Event 1 start of conversion (DCAEVT1.soc)  adcstartModuleB=off  adcrequestEventB=First event  adcstartEventB=Counter equals to zero (CTR=Zero)  adcstartEventB_type2=Counter equals to zero (CTR=Zero)  intEn=off  intPrd=First event  intSel=Counter equals to zero (CTR=Zero)  intSel_type2=Counter equals to zero (CTR=Zero)  hrpe=off  enHRPWM=off  HRPWM_LoadMode=Counter equals to period (CTR=PRD)  HRPWM_CTLMode=Duty or Period control mode  HRPWM_EDGMode=Both edge  hrpeb=off  enHRPWMB=off  HRPWM_LoadModeB=Counter equals to zero (CTR=ZERO)  HRPWM_CTLModeB=Duty or Period control mode  HRPWM_EDGModeB=Both edge  enHRDBRED=off  enHRDBFED=off  enSFO=on  enautoconv=on  chopperEnable=off  chopperFrequency=1  chopperFirstwidth=1  chopperDuty=12.5%  tripZonesource=Specify via dialog  tzselOSHT1=off  tzselOSHT2=off  tzselOSHT3=off  tzselOSHDCAEV1=off  tzselOSHDCBEV1=off  tzselCBC1=off  tzselCBC2=off  tzselCBC3=off  tzselCBCDCAEV2=off  tzselCBCDCBEV2=off  tzselOSHT4=off  tzselOSHT5=off  tzselOSHT6=off  tzselCBC4=off  tzselCBC5=off  tzselCBC6=off  enTzOstIntr=off  enTzCbcIntr=off  enTzDCAEVT1Intr=off  enTzDCAEVT2Intr=off  enTzDCBEVT1Intr=off  enTzDCBEVT2Intr=off  ePWMxAforced=No action  ePWMxBforced=No action  DCAEVT1forced=No action  DCBEVT1forced=No action  DCAEVT2forced=No action  DCBEVT2forced=No action  dcah=Trip Zone 1 input (TZ1)  dcal=Trip Zone 2 input (TZ2)  dcbh=Trip Zone 1 input (TZ1)  dcbl=Trip Zone 2 input (TZ2)  dcah_type2=GPTRIP1SEL/(TZ1)  dcal_type2=GPTRIP2SEL/(TZ2)  dcbh_type2=GPTRIP1SEL/(TZ1)  dcbl_type2=GPTRIP2SEL/(TZ2)  gendcaevt1=Event disabled  gendcaevt2=Event disabled  gendcbevt1=Event disabled  gendcbevt2=Event disabled  dcaevt1src=DCAEVT1 with sync  dcaevt2src=DCAEVT2 with sync  dcbevt1src=DCBEVT1 with sync  dcbevt2src=DCBEVT2 with sync  pulsesel=Counter equals to zero (CTR=Zero)  blankinv=off  blankoffset=0  blankwidth=0  evsrcsel=Filtered version of DCAEVT1 (DCAEVT1FILT)  encape=off
  wires:
  Data Type Conversion/1 -> Bitwise Operator/1
  IQ_desired/1 -> Bias1/1
  Shift Arithmetic1/1 -> Mux/2
  Shift Arithmetic/1 -> Mux/1
  Mux/1 -> Data Type Conversion/1
  Demux/1 -> ePWM2/1
  Demux/2 -> ePWM2/2
  speed/1 -> Bias2/1
  Bias1/1 -> Shift Arithmetic1/1
  Bitwise Operator/1 -> Demux/1
  Bias2/1 -> Shift Arithmetic/1
